simulink model "simulink_aocs_spin"  (R2023b)
settings: Solver=VariableStepAuto  StartTime=0.0  StopTime=10.0  RelTol=1e-3
values from neighbouring files (symbols this model uses):
  A0 = [1 0 0; 0 0 1; 0 -1 0]*[0 0 1; 0 1 0; -1 0 0]    [planetary_phase_script.m]    (also in script_aocs.m = [0 0 1; 0 1 0; -1 0 0]; script_jupiter.m; simulation_inner1.m = A_b_n(:,:,end); srp_interplanetary.m = A_b_n(:,:,end))
  braccio_x = 2.7    [planetary_phase_script.m]    (also in script_aocs.m; script_jupiter.m; simulation_inner1.m; srp_interplanetary.m)
  braccio_y = 2.7    [planetary_phase_script.m]    (also in script_aocs.m; script_jupiter.m; simulation_inner1.m; srp_interplanetary.m)
  braccio_z = 3.2    [planetary_phase_script.m]    (also in script_aocs.m; script_jupiter.m; simulation_inner1.m; srp_interplanetary.m)
  gain_alphas = [-1000; -1000; -10]    [planetary_phase_script.m]    (also in script_aocs.m = -90; script_jupiter.m; simulation_inner1.m = [-100 -100 -1]'; srp_interplanetary.m = [-100 -100 -1]')
  gain_omega = -1    [planetary_phase_script.m]    (also in script_aocs.m = -9500; script_jupiter.m; simulation_inner1.m = -950; srp_interplanetary.m = -950)
  I = diag([11245.08 10044.71 17593.63])    [planetary_phase_script.m]    (also in script_aocs.m = [11245.08 0 0; 0 10044.71 0; 0 0 17593.63]; script_jupiter.m; simulation_inner1.m = [11245.08 0 0; 0 10044.71 0; 0 0 17593.63]; srp_interplanetary.m = [11245.08 0 0; 0 10044.71 0; 0 0 17593.63])
  I_inv = inv(I)    [planetary_phase_script.m]    (also in script_aocs.m; script_jupiter.m; simulation_inner1.m; srp_interplanetary.m)
  spin_fin = spin(j,2) * 2*pi/60    [script_aocs.m]
  t_s = 1    [script_aocs.m]    (also in simulation_inner1.m; srp_interplanetary.m)
  toll = deg2rad(15)    [planetary_phase_script.m]    (also in script_aocs.m; script_jupiter.m; simulation_inner1.m; srp_interplanetary.m)
  w0 = [0 0 n]    [planetary_phase_script.m]    (also in script_aocs.m = [0 0 spin_0]; script_jupiter.m; simulation_inner1.m = w(:,end); srp_interplanetary.m = w(:,end))
libraries: simulink x3, matrix_library x1
settings Model: SimulationMode=accelerator  Creator=paolo  LastModifiedBy=paolo

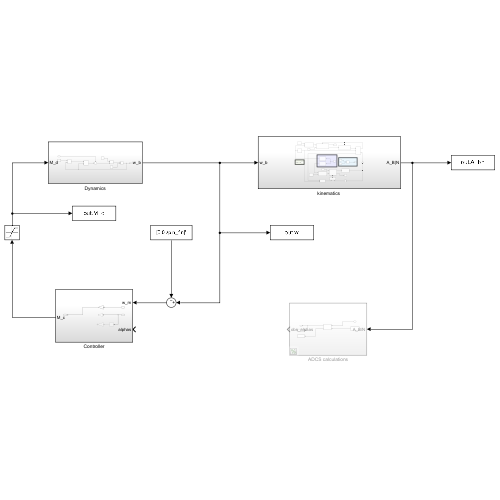
[thumbnail: Simulink's stored preview of the top-level diagram]
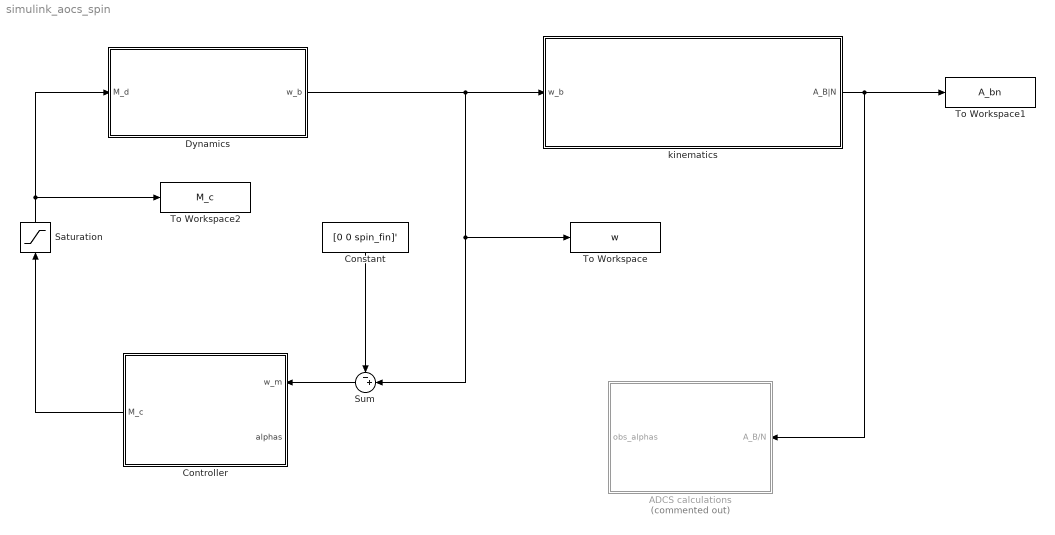
== system simulink_aocs_spin ==
  ADCS calculations : Subsystem  Commented=on
  Constant : Constant  Value=[0 0 spin_fin]'
  Controller : Subsystem
  Dynamics : Subsystem
  Saturation : Saturate  UpperLimit=5*[braccio_x braccio_y braccio_z]'  LowerLimit=-5*[braccio_x braccio_y braccio_z]'
  Sum : Sum  Inputs=-+|
  To Workspace : ToWorkspace  VariableName=w  SampleTime=-1
  To Workspace1 : ToWorkspace  VariableName=A_bn  SampleTime=-1
  To Workspace2 : ToWorkspace  VariableName=M_c  SampleTime=-1
  "kinematics " : Subsystem
  wires:
  "kinematics "/1(A_B|N) -> To Workspace1/1, ADCS calculations/1(" A_B/N")
  Saturation/1 -> Dynamics/1(M_d), To Workspace2/1
  Sum/1 -> Controller/1(w_m)
  Constant/1 -> Sum/1
  Dynamics/1(w_b) -> "kinematics "/1(w_b), To Workspace/1, Sum/2
  Controller/1(M_c) -> Saturation/1

== system simulink_aocs_spin/ADCS calculations ==
  " A_B/N" : Inport
  Error determination1 : Subsystem
  To Workspace10 : ToWorkspace  VariableName=alphas  SampleTime=-1
  To Workspace2 : ToWorkspace  VariableName=error_matrix  SampleTime=-1
  targeting attitude : Subsystem
  obs_alphas : Outport
  wires:
  Error determination1/2(Error Matrix) -> To Workspace2/1
  Error determination1/1(alphas) -> To Workspace10/1, obs_alphas/1
  targeting attitude/1(target) -> Error determination1/2(target)
  " A_B/N"/1 -> Error determination1/1(sensed A_b|n)

== system simulink_aocs_spin/Controller ==
  w_m : Inport
  alphas : Inport  Port=2
  Gain1 : Gain  Commented=on  Gain=-0.0075
  Gain3 : Gain  Gain=gain_omega
  Gain4 : Gain  Commented=on  Gain=gain_alphas
  Integrator : Integrator  Commented=on
  M_c : Outport
  wires:
  Gain3/1 -> M_c/1
  w_m/1 -> Gain3/1  "w_m"
  alphas/1 -> Integrator/1, Gain4/1  "alphas"
  Integrator/1 -> Gain1/1

== system simulink_aocs_spin/Dynamics ==
  M_d : Inport
  Add : Sum  Inputs=++|
  Constant : Constant  Value=I_inv
  Constant1 : Constant  Value=I
  Constant2 : Constant  Value=w0
  Cross Product : matrix_library/Cross Product
  Integrator : Integrator  InitialConditionSource=external
  Product3 : Product  Multiplication=Matrix(*)
  Product4 : Product  Multiplication=Matrix(*)
  w_b : Outport
  wires:
  Constant2/1 -> Integrator/2
  Integrator/1 -> Cross Product/2, Product3/2, w_b/1
  Constant1/1 -> Product3/1
  Product3/1 -> Cross Product/1
  Cross Product/1 -> Add/2
  Constant/1 -> Product4/1
  Product4/1 -> Integrator/1
  Add/1 -> Product4/2
  M_d/1 -> Add/1

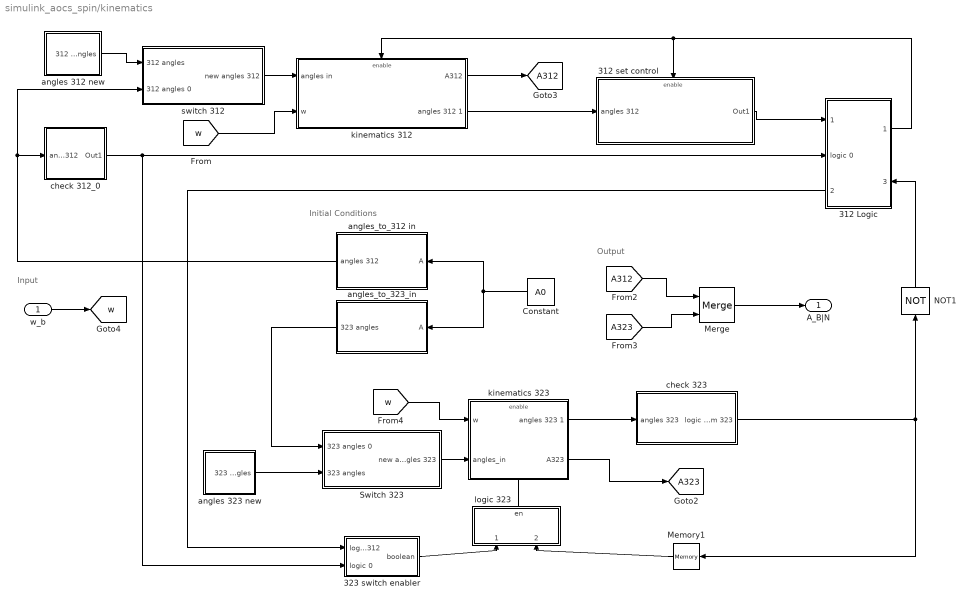
== system simulink_aocs_spin/kinematics  ==
  note: Initial Conditions
  note: Input
  note: Output
  w_b : Inport
  312 Logic : Subsystem
      settings: PortSchema="{\"entries\":[{\"content\":{\"sides\":[{\"content\":{\"connectorIds\":[\"In1\",\"In2\",\"Out2\"]},\"type\":\"ConnectorPlacement.EquallySpacedRectSide\",\"uuid\":\"bbe9512c-7163-4fef-b9d1-43cb9aeff445\"},{\"content\":{\"connectorIds\":[\"Out1\",\"In3\"],\"side\":\"RIGHT\"},\"type\":\"ConnectorPlacement.EquallySpacedRectSide\",\"uuid\":\"277562d8-09f7-4de0-8511-9dc3831eb0dd\"},{\"content\":{\"side\":\"TOP\"},\"type\":\"ConnectorPlacement.EquallySpacedRectSide\",\"uuid\":\"e92148c3-32f1-4524-99fb-140743ec3546\"},{\"content\":{\"side\":\"BOTTOM\"},\"type\":\"ConnectorPlacement.EquallySpacedRectSide\",\"uuid\":\"83e80a71-3551-431b-aa8d-7f5ff14dcfcb\"}]},\"type\":\"ConnectorPlacement.EquallySpacedConnector\",\"uuid\":\"c3d5c0ca-8775-4917-b094-b0cdc270e969\"}],\"packageUris\":[\"http://schema.mathworks.com/mf0/Connector/R2020b\"],\"version\":\"1.0\"}"
  312 set control : Subsystem
  323 switch enabler : Subsystem
  Constant : Constant  Value=A0
  Memory1 : Memory
  Merge : Merge
  NOT1 : Logic  Operator=NOT  IconShape=distinctive  AllPortsSameDT=off  OutDataTypeStr=boolean
  Switch 323 : Subsystem
  angles 312 new : Subsystem
  angles 323 new : Subsystem
  angles_to_312 in : Subsystem
  angles_to_323_in : Subsystem
  check 312_0 : Subsystem
      settings: PortSchema="{\"entries\":[{\"content\":{\"sides\":[{\"content\":{},\"type\":\"ConnectorPlacement.EquallySpacedRectSide\",\"uuid\":\"ce510fac-c30a-4239-a3ca-34d3b3a25917\"},{\"content\":{\"side\":\"RIGHT\"},\"type\":\"ConnectorPlacement.EquallySpacedRectSide\",\"uuid\":\"eef8e0af-d591-4c9d-a699-4633d685d136\"},{\"content\":{\"connectorIds\":[\"Out1\"],\"side\":\"TOP\"},\"type\":\"ConnectorPlacement.EquallySpacedRectSide\",\"uuid\":\"fcaa08d0-a3a1-4dce-b64a-8b5dfd06733d\"},{\"content\":{\"connectorIds\":[\"In1\"],\"side\":\"BOTTOM\"},\"type\":\"ConnectorPlacement.EquallySpacedRectSide\",\"uuid\":\"e9ea2ab9-2ba0-4219-9d61-f42bbc501f13\"}]},\"type\":\"ConnectorPlacement.EquallySpacedConnector\",\"uuid\":\"4537d4ba-38a8-4a93-90f3-8d5d5085984b\"}],\"packageUris\":[\"http://schema.mathworks.com/mf0/Connector/R2020b\"],\"version\":\"1.0\"}"
  check 323 : Subsystem
      settings: PortSchema="{\"entries\":[{\"content\":{\"sides\":[{\"content\":{},\"type\":\"ConnectorPlacement.EquallySpacedRectSide\",\"uuid\":\"ce510fac-c30a-4239-a3ca-34d3b3a25917\"},{\"content\":{\"side\":\"RIGHT\"},\"type\":\"ConnectorPlacement.EquallySpacedRectSide\",\"uuid\":\"eef8e0af-d591-4c9d-a699-4633d685d136\"},{\"content\":{\"connectorIds\":[\"Out1\"],\"side\":\"TOP\"},\"type\":\"ConnectorPlacement.EquallySpacedRectSide\",\"uuid\":\"fcaa08d0-a3a1-4dce-b64a-8b5dfd06733d\"},{\"content\":{\"connectorIds\":[\"In1\"],\"side\":\"BOTTOM\"},\"type\":\"ConnectorPlacement.EquallySpacedRectSide\",\"uuid\":\"e9ea2ab9-2ba0-4219-9d61-f42bbc501f13\"}]},\"type\":\"ConnectorPlacement.EquallySpacedConnector\",\"uuid\":\"4537d4ba-38a8-4a93-90f3-8d5d5085984b\"}],\"packageUris\":[\"http://schema.mathworks.com/mf0/Connector/R2020b\"],\"version\":\"1.0\"}"
  kinematics 312 : Subsystem
  kinematics 323 : Subsystem
  logic 323 : Subsystem
  switch 312 : Subsystem
  A_B|N : Outport
  tag scope: A312=global, A323=global, w=global
  wires:
  kinematics 323/2(A323) -> [A323]
  Constant/1 -> angles_to_323_in/1(A), angles_to_312 in/1(A)
  323 switch enabler/1(boolean) -> logic 323/1(boolean from 312)
  logic 323/1(en) -> kinematics 323/Enable
  kinematics 312/2(angles 312 1) -> 312 set control/1(angles 312)
  check 312_0/1(Out1) -> 323 switch enabler/2(logic 0), 312 Logic/2(logic 0)
  [w] -> kinematics 323/1(w)
  angles_to_312 in/1(angles 312) -> switch 312/2(312 angles 0), check 312_0/1(angles 312)
  Memory1/1 -> logic 323/2(boolean from 323)
  w_b/1 -> [w]
  kinematics 323/1(angles 323 1) -> check 323/1(angles 323)
  kinematics 312/1(A312) -> [A312]
  switch 312/1(new angles 312) -> kinematics 312/1(angles in)
  Merge/1 -> A_B|N/1
  Switch 323/1(new angles 323) -> kinematics 323/2(angles_in)
  check 323/1(logic from 323) -> NOT1/1, Memory1/1
  angles 323 new/1(323 angles) -> Switch 323/2(323 angles)
  angles 312 new/1(312 angles) -> switch 312/1(312 angles)
  [w] -> kinematics 312/2(w)
  angles_to_323_in/1(323 angles) -> Switch 323/1(323 angles 0)
  [A323] -> Merge/2
  [A312] -> Merge/1
  312 Logic/1(logic to 312) -> kinematics 312/Enable, 312 set control/Enable
  312 set control/1(Out1) -> 312 Logic/1(logic from 312)
  NOT1/1 -> 312 Logic/3(logic from 323)
  312 Logic/2(logic to 323) -> 323 switch enabler/1(logic from 312)

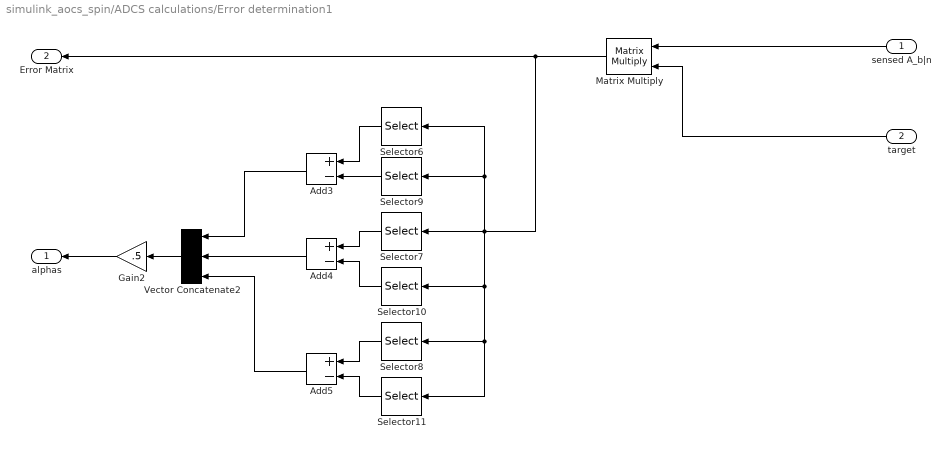
== system simulink_aocs_spin/ADCS calculations/Error determination1 ==
  sensed A_b|n : Inport
  target : Inport  Port=2
  Add3 : Sum  Inputs=+-
  Add4 : Sum  Inputs=+-
  Add5 : Sum  Inputs=+-
  Gain2 : Gain  Gain=.5
  Matrix Multiply : Product  Multiplication=Matrix(*)
  Selector10 : Selector  NumberOfDimensions=2  InputPortWidth=3  IndexOptions=Index vector (dialog),Index vector (dialog)  Indices=1,3  OutputSizes=1,1
  Selector11 : Selector  NumberOfDimensions=2  InputPortWidth=3  IndexOptions=Index vector (dialog),Index vector (dialog)  Indices=2,1  OutputSizes=1,1
  Selector6 : Selector  NumberOfDimensions=2  InputPortWidth=3  IndexOptions=Index vector (dialog),Index vector (dialog)  Indices=2,3  OutputSizes=1,1
  Selector7 : Selector  NumberOfDimensions=2  InputPortWidth=3  IndexOptions=Index vector (dialog),Index vector (dialog)  Indices=3,1  OutputSizes=1,1
  Selector8 : Selector  NumberOfDimensions=2  InputPortWidth=3  IndexOptions=Index vector (dialog),Index vector (dialog)  Indices=1,2  OutputSizes=1,1
  Selector9 : Selector  NumberOfDimensions=2  InputPortWidth=3  IndexOptions=Index vector (dialog),Index vector (dialog)  Indices=3,2  OutputSizes=1,1
  Vector Concatenate2 : Concatenate  NumInputs=3
  alphas : Outport
  Error Matrix : Outport  Port=2
  wires:
  Gain2/1 -> alphas/1
  Add4/1 -> Vector Concatenate2/2
  Selector6/1 -> Add3/1
  Selector11/1 -> Add5/2
  Vector Concatenate2/1 -> Gain2/1
  Add3/1 -> Vector Concatenate2/1
  Selector7/1 -> Add4/1
  Selector10/1 -> Add4/2
  Matrix Multiply/1 -> Selector7/1, Selector10/1, Selector11/1, Selector8/1, Selector9/1, Selector6/1, Error Matrix/1
  Selector8/1 -> Add5/1
  Selector9/1 -> Add3/2
  Add5/1 -> Vector Concatenate2/3
  sensed A_b|n/1 -> Matrix Multiply/1
  target/1 -> Matrix Multiply/2

== system simulink_aocs_spin/ADCS calculations/targeting attitude ==
  Constant1 : Constant  Value=[0 0 -1; 0 1 0; 1 0 0]
  Matrix Multiply : Product  Multiplication=Matrix(*)
  Rotation matrix n : Subsystem
  target : Outport
  wires:
  Matrix Multiply/1 -> target/1
  Constant1/1 -> Matrix Multiply/1
  Rotation matrix n/1(Target matrix) -> Matrix Multiply/2

== system simulink_aocs_spin/kinematics /312 Logic ==
  logic from 312 : Inport
  logic 0 : Inport  Port=2
  logic from 323 : Inport  Port=3
  Memory : Memory  InheritSampleTime=on
  Subsystem3 : Subsystem
  switch enabler 312 : Subsystem
  logic to 312 : Outport
  logic to 323 : Outport  Port=2
  wires:
  Subsystem3/1(Out1) -> Memory/1
  logic 0/1 -> switch enabler 312/2(In2)
  Memory/1 -> switch enabler 312/1(In1), Subsystem3/3(In3), logic to 323/1
  logic from 323/1 -> Subsystem3/2(In2)
  switch enabler 312/1(Out1) -> logic to 312/1
  logic from 312/1 -> Subsystem3/1(In1)

== system simulink_aocs_spin/kinematics /312 set control ==
  angles 312 : Inport
  Enable : EnablePort
  Check Static Range : simulink/Model Verification/Check  Static Range  Description=-pi/2+toll <= u <= pi/2 - toll  max=pi/2 - toll  max_included=on  min=-pi/2+toll  min_included=on  enabled=off  stopWhenAssertionFail=off  export=on  icon=graphic
  Selector : Selector  InputPortWidth=3  IndexOptions=Index vector (dialog)  Indices=2  OutputSizes=1
  Out1 : Outport
  wires:
  Check Static Range/1 -> Out1/1
  angles 312/1 -> Selector/1
  Selector/1 -> Check Static Range/1

== system simulink_aocs_spin/kinematics /323 switch enabler ==
  logic from 312 : Inport
  logic 0 : Inport  Port=2
  Clock2 : Clock
  NOT : Logic  Operator=NOT  IconShape=distinctive  AllPortsSameDT=off  OutDataTypeStr=boolean
  Switch2 : Switch  Criteria=u2 > Threshold  SaturateOnIntegerOverflow=off  InputSameDT=off
  boolean : Outport
  wires:
  Switch2/1 -> NOT/1
  logic 0/1 -> Switch2/3
  Clock2/1 -> Switch2/2
  logic from 312/1 -> Switch2/1
  NOT/1 -> boolean/1

== system simulink_aocs_spin/kinematics /Switch 323 ==
  323 angles 0 : Inport
  323 angles : Inport  Port=2
  Clock3 : Clock
  Switch3 : Switch  Criteria=u2 > Threshold  SaturateOnIntegerOverflow=off  InputSameDT=off
  new angles 323 : Outport
  wires:
  Clock3/1 -> Switch3/2
  323 angles 0/1 -> Switch3/3
  323 angles/1 -> Switch3/1
  Switch3/1 -> new angles 323/1

== system simulink_aocs_spin/kinematics /angles 312 new ==
  A323 matrix : Subsystem
  angles_to_312 : Subsystem
  312 angles : Outport
  wires:
  [phi323] -> A323 matrix/1(phi)
  [theta323] -> A323 matrix/2(theta)
  [psi323] -> A323 matrix/3(psi)
  angles_to_312/1(312 angles) -> 312 angles/1
  A323 matrix/1(A323) -> angles_to_312/1(A323)

== system simulink_aocs_spin/kinematics /angles 323 new ==
  Rotation 312 matrix2 : Subsystem
  angles_to_323 : Subsystem
  323 angles : Outport
  wires:
  [theta312] -> Rotation 312 matrix2/2(theta)
  [psi_312] -> Rotation 312 matrix2/3(psi)
  Rotation 312 matrix2/1(A312) -> angles_to_323/1(A312)
  [phi312] -> Rotation 312 matrix2/1(phi)
  angles_to_323/1(323 angles) -> 323 angles/1

== system simulink_aocs_spin/kinematics /angles_to_312 in ==
  A : Inport
  Asin : Trigonometry  Operator=asin
  Atan1 : Trigonometry  Operator=atan2
  Atan2 : Trigonometry  Operator=atan2
  Gain : Gain  Gain=-1
  Gain1 : Gain  Gain=-1
  Mux : Mux  Inputs=3
  Selector : Selector  NumberOfDimensions=2  InputPortWidth=3  IndexOptions=Index vector (dialog),Index vector (dialog)  Indices=2,1  OutputSizes=1,1
  Selector1 : Selector  NumberOfDimensions=2  InputPortWidth=3  IndexOptions=Index vector (dialog),Index vector (dialog)  Indices=2,2  OutputSizes=1,1
  Selector2 : Selector  NumberOfDimensions=2  InputPortWidth=3  IndexOptions=Index vector (dialog),Index vector (dialog)  Indices=2,3  OutputSizes=1,1
  Selector3 : Selector  NumberOfDimensions=2  InputPortWidth=3  IndexOptions=Index vector (dialog),Index vector (dialog)  Indices=1,3  OutputSizes=1,1
  Selector4 : Selector  NumberOfDimensions=2  InputPortWidth=3  IndexOptions=Index vector (dialog),Index vector (dialog)  Indices=3,3  OutputSizes=1,1
  angles 312 : Outport
  wires:
  Selector/1 -> Gain/1
  Gain/1 -> Atan2/1
  Selector1/1 -> Atan2/2
  Selector2/1 -> Asin/1
  Atan2/1 -> Mux/1
  Asin/1 -> Mux/2
  Mux/1 -> angles 312/1
  A/1 -> Selector3/1, Selector4/1, Selector2/1, Selector/1, Selector1/1
  Selector3/1 -> Gain1/1
  Gain1/1 -> Atan1/1
  Selector4/1 -> Atan1/2
  Atan1/1 -> Mux/3

== system simulink_aocs_spin/kinematics /angles_to_323_in ==
  A : Inport
  Asin : Trigonometry  Operator=acos
  Atan1 : Trigonometry  Operator=atan2
  Atan2 : Trigonometry  Operator=atan2
  Gain2 : Gain  Gain=-1
  Mux : Mux  Inputs=3
  Selector : Selector  NumberOfDimensions=2  InputPortWidth=3  IndexOptions=Index vector (dialog),Index vector (dialog)  Indices=3,2  OutputSizes=1,1
  Selector1 : Selector  NumberOfDimensions=2  InputPortWidth=3  IndexOptions=Index vector (dialog),Index vector (dialog)  Indices=3,1  OutputSizes=1,1
  Selector2 : Selector  NumberOfDimensions=2  InputPortWidth=3  IndexOptions=Index vector (dialog),Index vector (dialog)  Indices=3,3  OutputSizes=1,1
  Selector3 : Selector  NumberOfDimensions=2  InputPortWidth=3  IndexOptions=Index vector (dialog),Index vector (dialog)  Indices=2,3  OutputSizes=1,1
  Selector4 : Selector  NumberOfDimensions=2  InputPortWidth=3  IndexOptions=Index vector (dialog),Index vector (dialog)  Indices=1,3  OutputSizes=1,1
  323 angles : Outport
  wires:
  Gain2/1 -> Atan1/2
  Selector1/1 -> Atan2/2
  Selector2/1 -> Asin/1
  Selector/1 -> Atan2/1
  A/1 -> Selector2/1, Selector4/1, Selector3/1, Selector1/1, Selector/1
  Atan1/1 -> Mux/3
  Atan2/1 -> Mux/1
  Selector4/1 -> Gain2/1
  Selector3/1 -> Atan1/1
  Asin/1 -> Mux/2
  Mux/1 -> 323 angles/1

== system simulink_aocs_spin/kinematics /check 312_0 ==
  angles 312 : Inport
  Check Static Range : simulink/Model Verification/Check  Static Range  Description=-pi/2+toll <= u <= pi/2 - toll  max=pi/2 - toll  max_included=on  min=-pi/2+toll  min_included=on  enabled=off  stopWhenAssertionFail=off  export=on  icon=graphic
  Data Type Conversion : DataTypeConversion  OutDataTypeStr=boolean  SaturateOnIntegerOverflow=off  RndMeth=Floor
  Selector : Selector  InputPortWidth=3  IndexOptions=Index vector (dialog)  Indices=[2]  OutputSizes=1
  Out1 : Outport
  wires:
  angles 312/1 -> Selector/1
  Selector/1 -> Check Static Range/1
  Check Static Range/1 -> Data Type Conversion/1
  Data Type Conversion/1 -> Out1/1

== system simulink_aocs_spin/kinematics /check 323 ==
  angles 323 : Inport
  Check Static Range : simulink/Model Verification/Check  Static Range  Description=toll <= u <= pi - toll  max=pi - toll  max_included=on  min=toll  min_included=on  enabled=off  stopWhenAssertionFail=off  export=on  icon=graphic
  Selector : Selector  InputPortWidth=3  IndexOptions=Index vector (dialog)  Indices=2  OutputSizes=1
  logic from 323 : Outport
  wires:
  Check Static Range/1 -> logic from 323/1
  Selector/1 -> Check Static Range/1
  angles 323/1 -> Selector/1

== system simulink_aocs_spin/kinematics /kinematics 312 ==
  angles in : Inport
  w : Inport  Port=2
  Enable : EnablePort  StatesWhenEnabling=reset  ShowOutputPort=on
  Kinematics 312 : Subsystem
      settings: PortSchema="{\"entries\":[{\"content\":{\"sides\":[{\"content\":{\"connectorIds\":[\"In1\",\"In2\"]},\"type\":\"ConnectorPlacement.EquallySpacedRectSide\",\"uuid\":\"4fd6e809-7da2-4d51-96c7-4627657bb0a7\"},{\"content\":{\"connectorIds\":[\"Out1\"],\"side\":\"RIGHT\"},\"type\":\"ConnectorPlacement.EquallySpacedRectSide\",\"uuid\":\"c66e7720-5f48-4c1c-aaff-2c7b43e45843\"},{\"content\":{\"connectorIds\":[\"In3\"],\"side\":\"TOP\"},\"type\":\"ConnectorPlacement.EquallySpacedRectSide\",\"uuid\":\"5add9d35-dacd-40f3-b2c8-04b7016dc331\"}]},\"type\":\"ConnectorPlacement.EquallySpacedConnector\",\"uuid\":\"f50f8b24-6836-47e2-b898-11b49150a1de\"}],\"packageUris\":[\"http://schema.mathworks.com/mf0/Connector/R2020b\"],\"version\":\"1.0\"}"
  Rotation 312 matrix1 : Subsystem
  A312 : Outport
  angles 312 1 : Outport  Port=2
  wires:
  Rotation 312 matrix1/1(A312) -> A312/1
  Kinematics 312/1(angles) -> Rotation 312 matrix1/1(angles), angles 312 1/1
  angles in/1 -> Kinematics 312/2(angles in)
  w/1 -> Kinematics 312/1(w)
  Enable/1 -> Kinematics 312/3(enabler)

== system simulink_aocs_spin/kinematics /kinematics 323 ==
  w : Inport
  angles_in : Inport  Port=2
  Enable : EnablePort  StatesWhenEnabling=reset  ShowOutputPort=on
  " kinematics 323" : Subsystem
      settings: PortSchema="{\"entries\":[{\"content\":{\"sides\":[{\"content\":{\"connectorIds\":[\"In1\",\"In2\"]},\"type\":\"ConnectorPlacement.EquallySpacedRectSide\",\"uuid\":\"4fd6e809-7da2-4d51-96c7-4627657bb0a7\"},{\"content\":{\"connectorIds\":[\"Out1\"],\"side\":\"RIGHT\"},\"type\":\"ConnectorPlacement.EquallySpacedRectSide\",\"uuid\":\"c66e7720-5f48-4c1c-aaff-2c7b43e45843\"},{\"content\":{\"connectorIds\":[\"In3\"],\"side\":\"TOP\"},\"type\":\"ConnectorPlacement.EquallySpacedRectSide\",\"uuid\":\"5add9d35-dacd-40f3-b2c8-04b7016dc331\"}]},\"type\":\"ConnectorPlacement.EquallySpacedConnector\",\"uuid\":\"f50f8b24-6836-47e2-b898-11b49150a1de\"}],\"packageUris\":[\"http://schema.mathworks.com/mf0/Connector/R2020b\"],\"version\":\"1.0\"}"
  A323 matrix1 : Subsystem
  angles 323 1 : Outport
  A323 : Outport  Port=2
  wires:
  angles_in/1 -> " kinematics 323"/1(angles_in)
  w/1 -> " kinematics 323"/2(w)
  A323 matrix1/1(A323) -> A323/1
  " kinematics 323"/1(angles) -> angles 323 1/1, A323 matrix1/1(angles)
  Enable/1 -> " kinematics 323"/3(enable)

== system simulink_aocs_spin/kinematics /logic 323 ==
  boolean from 312 : Inport
  boolean from 323 : Inport  Port=2
  AND : Logic  IconShape=distinctive  AllPortsSameDT=off  OutDataTypeStr=boolean
  Clock3 : Clock
  Memory : Memory
  Subsystem4 : Subsystem
  Switch3 : Switch  Criteria=u2 > Threshold  SaturateOnIntegerOverflow=off  InputSameDT=off
  en : Outport
  wires:
  Switch3/1 -> en/1, Memory/1
  Clock3/1 -> Switch3/2
  boolean from 323/1 -> Subsystem4/1(In2), AND/1
  boolean from 312/1 -> Subsystem4/3(In4), Switch3/3, AND/2
  Subsystem4/1(Out1) -> Switch3/1
  AND/1 -> Subsystem4/2(In1)
  Memory/1 -> Subsystem4/4(In3)

== system simulink_aocs_spin/kinematics /switch 312 ==
  312 angles : Inport
  312 angles 0 : Inport  Port=2
  Clock : Clock
  Switch : Switch  Criteria=u2 > Threshold  SaturateOnIntegerOverflow=off  InputSameDT=off
  new angles 312 : Outport
  wires:
  Switch/1 -> new angles 312/1
  312 angles/1 -> Switch/1
  Clock/1 -> Switch/2
  312 angles 0/1 -> Switch/3

== system simulink_aocs_spin/ADCS calculations/targeting attitude/Rotation matrix n ==
  Constant : Constant  Value=0
  Constant1 : Constant
  Cos : Trigonometry  Operator=cos
  Digital Clock : DigitalClock  SampleTime=t_s
  Gain : Gain  Gain=spin_fin
  Gain1 : Gain
  Gain2 : Gain  Gain=-1
  Sin : Trigonometry
  Target : Concatenate  NumInputs=3  Mode=Multidimensional array  ConcatenateDimension=2
  Vector Concatenate : Concatenate  NumInputs=3
  Vector Concatenate1 : Concatenate  NumInputs=3
  Vector Concatenate2 : Concatenate  NumInputs=3
  Target matrix : Outport
  wires:
  Vector Concatenate/1 -> Target/1
  Sin/1 -> Gain2/1, Gain1/1
  Cos/1 -> Vector Concatenate2/1, Vector Concatenate1/2
  Digital Clock/1 -> Gain/1
  Gain/1 -> Cos/1, Sin/1
  Constant/1 -> Vector Concatenate/1, Vector Concatenate2/3, Vector Concatenate1/3, Vector Concatenate/2
  Vector Concatenate2/1 -> Target/3
  Vector Concatenate1/1 -> Target/2
  Target/1 -> Target matrix/1
  Constant1/1 -> Vector Concatenate/3
  Gain1/1 -> Vector Concatenate1/1
  Gain2/1 -> Vector Concatenate2/2

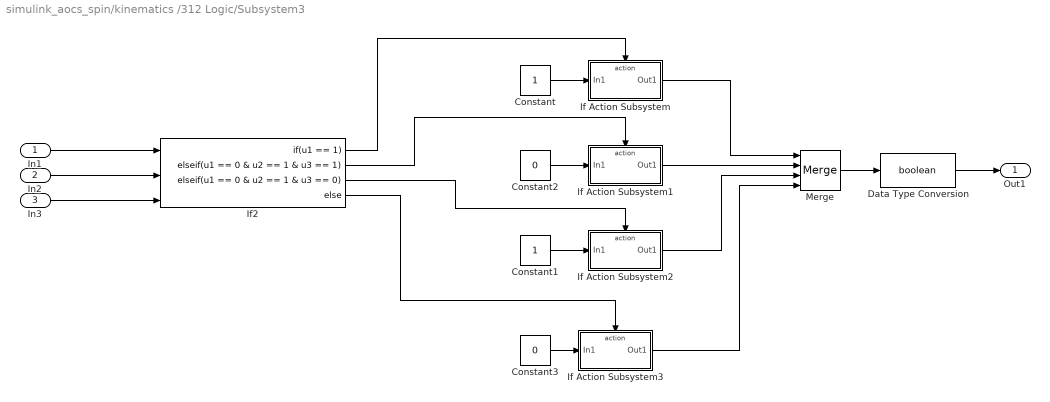
== system simulink_aocs_spin/kinematics /312 Logic/Subsystem3 ==
  In1 : Inport
  In2 : Inport  Port=2
  In3 : Inport  Port=3
  Constant : Constant
  Constant1 : Constant
  Constant2 : Constant  Value=0
  Constant3 : Constant  Value=0
  Data Type Conversion : DataTypeConversion  OutDataTypeStr=boolean  SaturateOnIntegerOverflow=off  RndMeth=Floor
  If Action Subsystem : Subsystem  TreatAsAtomicUnit=on
  If Action Subsystem1 : Subsystem  TreatAsAtomicUnit=on
  If Action Subsystem2 : Subsystem  TreatAsAtomicUnit=on
  If Action Subsystem3 : Subsystem  TreatAsAtomicUnit=on
  If2 : If  NumInputs=3  IfExpression=u1 == 1  ElseIfExpressions=u1 == 0 & u2 == 1 & u3 == 1, u1 == 0 & u2 == 1 & u3 == 0
  Merge : Merge  Inputs=4
  Out1 : Outport
  wires:
  In2/1 -> If2/2
  In1/1 -> If2/1
  In3/1 -> If2/3
  If2/1 -> If Action Subsystem/Action
  If2/2 -> If Action Subsystem1/Action
  If2/3 -> If Action Subsystem2/Action
  If2/4 -> If Action Subsystem3/Action
  Constant/1 -> If Action Subsystem/1(In1)
  Constant1/1 -> If Action Subsystem2/1(In1)
  Constant2/1 -> If Action Subsystem1/1(In1)
  Constant3/1 -> If Action Subsystem3/1(In1)
  If Action Subsystem/1(Out1) -> Merge/1
  If Action Subsystem1/1(Out1) -> Merge/2
  If Action Subsystem2/1(Out1) -> Merge/3
  If Action Subsystem3/1(Out1) -> Merge/4
  Merge/1 -> Data Type Conversion/1
  Data Type Conversion/1 -> Out1/1

== system simulink_aocs_spin/kinematics /312 Logic/switch enabler 312 ==
  In1 : Inport
  In2 : Inport  Port=2
  Clock1 : Clock
  Switch1 : Switch  Criteria=u2 > Threshold  SaturateOnIntegerOverflow=off  InputSameDT=off
  Out1 : Outport
  wires:
  In2/1 -> Switch1/3
  Clock1/1 -> Switch1/2
  In1/1 -> Switch1/1
  Switch1/1 -> Out1/1

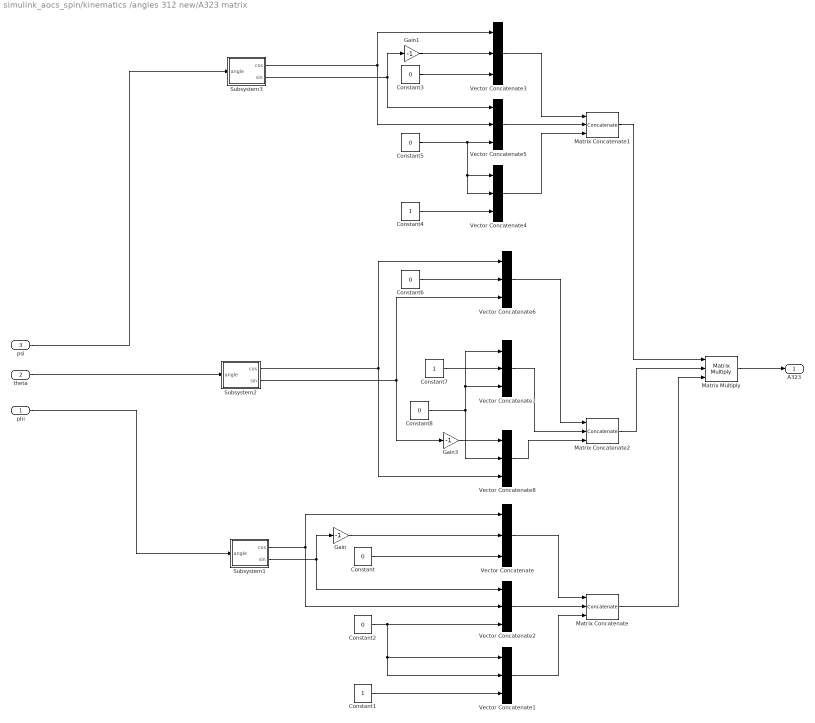
== system simulink_aocs_spin/kinematics /angles 312 new/A323 matrix ==
  phi : Inport
  theta : Inport  Port=2
  psi : Inport  Port=3
  Constant{,2..3,5..6,8} (6 alike) : Constant  Value=0
  Constant1 : Constant
  Constant4 : Constant
  Constant7 : Constant
  Gain : Gain  Gain=-1
  Gain1 : Gain  Gain=-1
  Gain3 : Gain  Gain=-1
  Matrix Concatenate : Concatenate  NumInputs=3  Mode=Multidimensional array  ConcatenateDimension=2
  Matrix Concatenate1 : Concatenate  NumInputs=3  Mode=Multidimensional array  ConcatenateDimension=2
  Matrix Concatenate2 : Concatenate  NumInputs=3  Mode=Multidimensional array  ConcatenateDimension=2
  Matrix Multiply : Product  Inputs=3  Multiplication=Matrix(*)
  Subsystem1 : Subsystem
  Subsystem2 : Subsystem
  Subsystem3 : Subsystem
  Vector Concatenate{,1..8} (9 alike) : Concatenate  NumInputs=3
  A323 : Outport
  wires:
  Subsystem1/2(sin) -> Gain/1, Vector Concatenate2/1
  Subsystem1/1(cos) -> Vector Concatenate2/2, Vector Concatenate/1
  Constant1/1 -> Vector Concatenate1/3
  Gain/1 -> Vector Concatenate/2
  Constant/1 -> Vector Concatenate/3
  Constant2/1 -> Vector Concatenate1/1, Vector Concatenate1/2, Vector Concatenate2/3
  Vector Concatenate/1 -> Matrix Concatenate/1
  Vector Concatenate2/1 -> Matrix Concatenate/2
  Vector Concatenate1/1 -> Matrix Concatenate/3
  Vector Concatenate4/1 -> Matrix Concatenate1/3
  Vector Concatenate5/1 -> Matrix Concatenate1/2
  Vector Concatenate3/1 -> Matrix Concatenate1/1
  Constant5/1 -> Vector Concatenate5/3, Vector Concatenate4/1, Vector Concatenate4/2
  Constant3/1 -> Vector Concatenate3/3
  Gain1/1 -> Vector Concatenate3/2
  Constant4/1 -> Vector Concatenate4/3
  Subsystem3/1(cos) -> Vector Concatenate3/1, Vector Concatenate5/2
  Subsystem3/2(sin) -> Vector Concatenate5/1, Gain1/1
  Matrix Concatenate2/1 -> Matrix Multiply/2
  Matrix Concatenate/1 -> Matrix Multiply/3
  Matrix Concatenate1/1 -> Matrix Multiply/1
  Matrix Multiply/1 -> A323/1
  Vector Concatenate6/1 -> Matrix Concatenate2/1
  Vector Concatenate7/1 -> Matrix Concatenate2/2
  Vector Concatenate8/1 -> Matrix Concatenate2/3
  Subsystem2/1(cos) -> Vector Concatenate8/3, Vector Concatenate6/1
  Constant6/1 -> Vector Concatenate6/2
  Subsystem2/2(sin) -> Vector Concatenate6/3, Gain3/1
  Constant7/1 -> Vector Concatenate7/2
  Constant8/1 -> Vector Concatenate7/1, Vector Concatenate7/3, Vector Concatenate8/2
  Gain3/1 -> Vector Concatenate8/1
  psi/1 -> Subsystem3/1(angle)
  theta/1 -> Subsystem2/1(angle)
  phi/1 -> Subsystem1/1(angle)

== system simulink_aocs_spin/kinematics /angles 312 new/angles_to_312 ==
  A323 : Inport
  Asin : Trigonometry  Operator=asin
  Atan1 : Trigonometry  Operator=atan2
  Atan2 : Trigonometry  Operator=atan2
  Gain : Gain  Gain=-1
  Gain1 : Gain  Gain=-1
  Mux : Mux  Inputs=3
  Selector : Selector  NumberOfDimensions=2  InputPortWidth=3  IndexOptions=Index vector (dialog),Index vector (dialog)  Indices=2,1  OutputSizes=1,1
  Selector1 : Selector  NumberOfDimensions=2  InputPortWidth=3  IndexOptions=Index vector (dialog),Index vector (dialog)  Indices=2,2  OutputSizes=1,1
  Selector2 : Selector  NumberOfDimensions=2  InputPortWidth=3  IndexOptions=Index vector (dialog),Index vector (dialog)  Indices=2,3  OutputSizes=1,1
  Selector3 : Selector  NumberOfDimensions=2  InputPortWidth=3  IndexOptions=Index vector (dialog),Index vector (dialog)  Indices=1,3  OutputSizes=1,1
  Selector4 : Selector  NumberOfDimensions=2  InputPortWidth=3  IndexOptions=Index vector (dialog),Index vector (dialog)  Indices=3,3  OutputSizes=1,1
  312 angles : Outport
  wires:
  Selector/1 -> Gain/1
  Gain/1 -> Atan2/1
  Selector1/1 -> Atan2/2
  Selector2/1 -> Asin/1
  Atan2/1 -> Mux/1
  Asin/1 -> Mux/2
  Mux/1 -> 312 angles/1
  A323/1 -> Selector/1, Selector1/1, Selector3/1, Selector4/1, Selector2/1
  Selector3/1 -> Gain1/1
  Gain1/1 -> Atan1/1
  Selector4/1 -> Atan1/2
  Atan1/1 -> Mux/3

== system simulink_aocs_spin/kinematics /angles 323 new/Rotation 312 matrix2 ==
  phi : Inport
  theta : Inport  Port=2
  psi : Inport  Port=3
  A312 conc : Concatenate  NumInputs=3  Mode=Multidimensional array  ConcatenateDimension=2
  Subsystem : Subsystem
  Subsystem1 : Subsystem
  Subsystem2 : Subsystem
  column 1 : Subsystem
  column 2 : Subsystem
  column 3 : Subsystem
  A312 : Outport
  wires:
  A312 conc/1 -> A312/1
  Subsystem/1(cos) -> column 2/1(phi), column 1/1(phi)
  column 3/1(Out1) -> A312 conc/3
  column 1/1(Out1) -> A312 conc/1
  Subsystem2/2(sin) -> column 3/4(psi2), column 2/6(psi2), column 1/6(psi2)
  column 2/1(Out1) -> A312 conc/2
  Subsystem2/1(cos) -> column 3/3(psi), column 1/5(psi), column 2/5(psi)
  Subsystem1/2(sin) -> column 2/4(theta2), column 1/4(theta2), column 3/2(theta2)
  Subsystem/2(sin) -> column 2/2(phi2), column 1/2(phi2)
  Subsystem1/1(cos) -> column 1/3(theta), column 3/1(theta), column 2/3(theta)
  phi/1 -> Subsystem/1(angle)
  theta/1 -> Subsystem1/1(angle)
  psi/1 -> Subsystem2/1(angle)

== system simulink_aocs_spin/kinematics /angles 323 new/angles_to_323 ==
  A312 : Inport
  Asin : Trigonometry  Operator=acos
  Atan1 : Trigonometry  Operator=atan2
  Atan2 : Trigonometry  Operator=atan2
  Gain2 : Gain  Gain=-1
  Mux : Mux  Inputs=3
  Selector : Selector  NumberOfDimensions=2  InputPortWidth=3  IndexOptions=Index vector (dialog),Index vector (dialog)  Indices=3,2  OutputSizes=1,1
  Selector1 : Selector  NumberOfDimensions=2  InputPortWidth=3  IndexOptions=Index vector (dialog),Index vector (dialog)  Indices=3,1  OutputSizes=1,1
  Selector2 : Selector  NumberOfDimensions=2  InputPortWidth=3  IndexOptions=Index vector (dialog),Index vector (dialog)  Indices=3,3  OutputSizes=1,1
  Selector3 : Selector  NumberOfDimensions=2  InputPortWidth=3  IndexOptions=Index vector (dialog),Index vector (dialog)  Indices=2,3  OutputSizes=1,1
  Selector4 : Selector  NumberOfDimensions=2  InputPortWidth=3  IndexOptions=Index vector (dialog),Index vector (dialog)  Indices=1,3  OutputSizes=1,1
  323 angles : Outport
  wires:
  Mux/1 -> 323 angles/1
  Asin/1 -> Mux/2
  Selector3/1 -> Atan1/1
  Selector4/1 -> Gain2/1
  Atan2/1 -> Mux/1
  Atan1/1 -> Mux/3
  A312/1 -> Selector/1, Selector1/1, Selector3/1, Selector4/1, Selector2/1
  Selector/1 -> Atan2/1
  Selector2/1 -> Asin/1
  Selector1/1 -> Atan2/2
  Gain2/1 -> Atan1/2

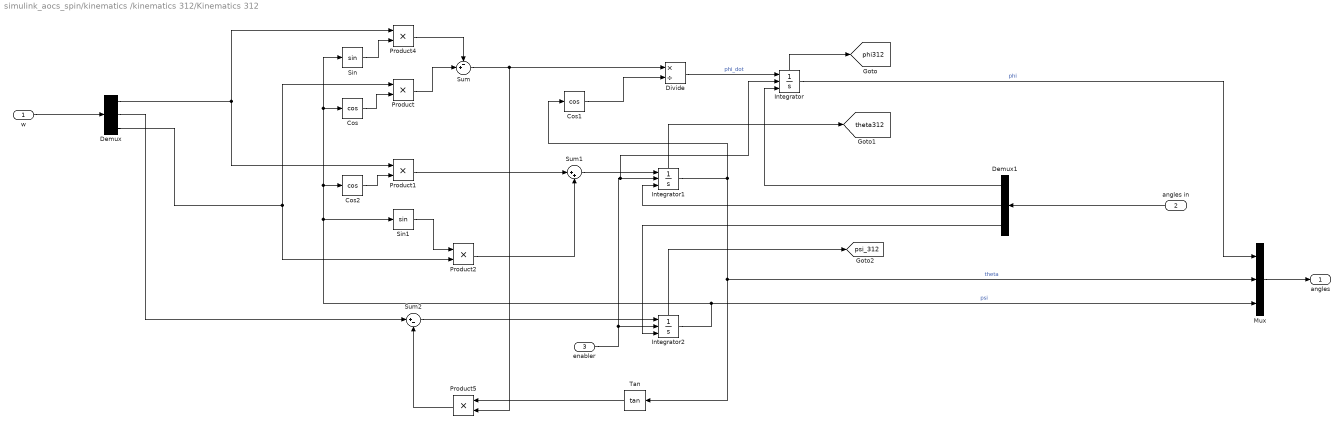
== system simulink_aocs_spin/kinematics /kinematics 312/Kinematics 312 ==
  w : Inport
  angles in : Inport  Port=2
  enabler : Inport  Port=3
  Cos : Trigonometry  Operator=cos
  Cos1 : Trigonometry  Operator=cos
  Cos2 : Trigonometry  Operator=cos
  Demux : Demux  Outputs=3
  Demux1 : Demux  Outputs=3
  Divide : Product  Inputs=*/
  Integrator : Integrator  ExternalReset=rising  InitialConditionSource=external  ShowStatePort=on
  Integrator1 : Integrator  ExternalReset=rising  InitialConditionSource=external  ShowStatePort=on
  Integrator2 : Integrator  ExternalReset=rising  InitialConditionSource=external  ShowStatePort=on  IgnoreLimit=on  ZeroCross=off
  Mux : Mux  Inputs=3
  Product{,1..2,4..5} (5 alike) : Product
  Sin : Trigonometry
  Sin1 : Trigonometry
  Sum : Sum  Inputs=-+|
  Sum1 : Sum  Inputs=|++
  Sum2 : Sum  Inputs=|+-
  Tan : Trigonometry  Operator=tan
  angles : Outport
  tag scope: phi312=global, psi_312=global, theta312=global
  wires:
  Integrator/1 -> Mux/1  "phi"
  Integrator1/1 -> Tan/1, Mux/2, Cos1/1  "theta"
  Integrator2/1 -> Sin/1, Cos/1, Cos2/1, Sin1/1, Mux/3  "psi"
  Cos/1 -> Product/2
  Demux/3 -> Product/1, Product2/2
  Product/1 -> Sum/2
  Sin/1 -> Product4/2
  Demux/1 -> Product4/1, Product1/1
  Cos1/1 -> Divide/2
  Divide/1 -> Integrator/1  "phi_dot"
  Cos2/1 -> Product1/2
  Product1/1 -> Sum1/1
  Sin1/1 -> Product2/1
  Product2/1 -> Sum1/2
  Sum1/1 -> Integrator1/1
  Product4/1 -> Sum/1
  Sum2/1 -> Integrator2/1
  Sum/1 -> Divide/1, Product5/2
  Tan/1 -> Product5/1
  Product5/1 -> Sum2/2
  Demux/2 -> Sum2/1
  w/1 -> Demux/1
  Mux/1 -> angles/1
  angles in/1 -> Demux1/1
  Demux1/1 -> Integrator/3
  Demux1/2 -> Integrator1/3
  Demux1/3 -> Integrator2/3
  enabler/1 -> Integrator/2, Integrator1/2, Integrator2/2
  Integrator/State -> [phi312]
  Integrator1/State -> [theta312]
  Integrator2/State -> [psi_312]

== system simulink_aocs_spin/kinematics /kinematics 312/Rotation 312 matrix1 ==
  angles : Inport
  A312 conc : Concatenate  NumInputs=3  Mode=Multidimensional array  ConcatenateDimension=2
  Demux : Demux  Outputs=3
  Subsystem : Subsystem
  Subsystem1 : Subsystem
  Subsystem2 : Subsystem
  column 1 : Subsystem
  column 2 : Subsystem
  column 3 : Subsystem
  A312 : Outport
  wires:
  angles/1 -> Demux/1
  Subsystem1/1(cos) -> column 2/3(theta), column 3/1(theta), column 1/3(theta)
  Subsystem/2(sin) -> column 1/2(phi2), column 2/2(phi2)
  Subsystem1/2(sin) -> column 3/2(theta2), column 1/4(theta2), column 2/4(theta2)
  Subsystem2/1(cos) -> column 2/5(psi), column 1/5(psi), column 3/3(psi)
  column 2/1(Out1) -> A312 conc/2
  Demux/2 -> Subsystem1/1(angle)
  Subsystem2/2(sin) -> column 1/6(psi2), column 2/6(psi2), column 3/4(psi2)
  Demux/3 -> Subsystem2/1(angle)
  column 1/1(Out1) -> A312 conc/1
  column 3/1(Out1) -> A312 conc/3
  Demux/1 -> Subsystem/1(angle)
  Subsystem/1(cos) -> column 1/1(phi), column 2/1(phi)
  A312 conc/1 -> A312/1

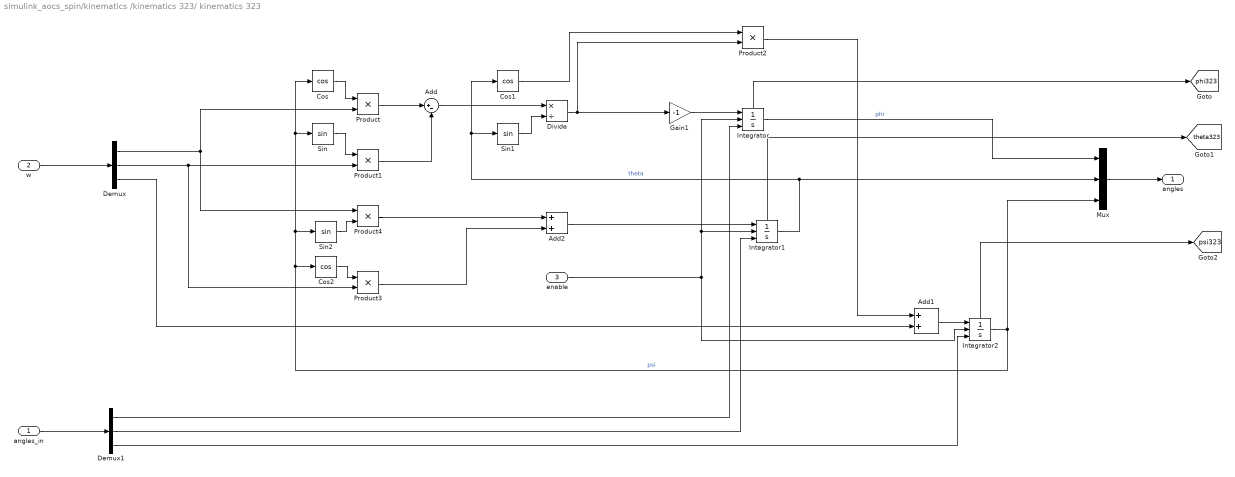
== system simulink_aocs_spin/kinematics /kinematics 323/ kinematics 323 ==
  angles_in : Inport
  w : Inport  Port=2
  enable : Inport  Port=3
  Add : Sum  Inputs=|+-
  Add1 : Sum
  Add2 : Sum
  Cos : Trigonometry  Operator=cos
  Cos1 : Trigonometry  Operator=cos
  Cos2 : Trigonometry  Operator=cos
  Demux : Demux  Outputs=3
  Demux1 : Demux  Outputs=3
  Divide : Product  Inputs=*/
  Gain1 : Gain  Gain=-1
  Integrator : Integrator  ExternalReset=rising  InitialConditionSource=external  ShowStatePort=on
  Integrator1 : Integrator  ExternalReset=rising  InitialConditionSource=external  ShowStatePort=on
  Integrator2 : Integrator  ExternalReset=rising  InitialConditionSource=external  ShowStatePort=on
  Mux : Mux  Inputs=3
  Product{,1..4} (5 alike) : Product
  Sin : Trigonometry
  Sin1 : Trigonometry
  Sin2 : Trigonometry
  angles : Outport
  tag scope: phi323=global, psi323=global, theta323=global
  wires:
  w/1 -> Demux/1
  Integrator2/1 -> Mux/3, Cos/1, Sin/1, Sin2/1, Cos2/1  "psi"
  Integrator1/1 -> Mux/2, Sin1/1, Cos1/1  "theta"
  Integrator/1 -> Mux/1  "phi"
  Demux/1 -> Product4/1, Product/2
  Cos/1 -> Product/1
  Product/1 -> Add/1
  Demux/2 -> Product3/2, Product1/2
  Sin/1 -> Product1/1
  Product1/1 -> Add/2
  Add/1 -> Divide/1
  Sin1/1 -> Divide/2
  Divide/1 -> Gain1/1, Product2/2
  Gain1/1 -> Integrator/1
  Cos1/1 -> Product2/1
  Demux/3 -> Add1/2
  Product2/1 -> Add1/1
  Add1/1 -> Integrator2/1
  Demux1/3 -> Integrator2/3
  Demux1/1 -> Integrator/3
  Cos2/1 -> Product3/1
  Sin2/1 -> Product4/2
  Product4/1 -> Add2/1
  Product3/1 -> Add2/2
  Add2/1 -> Integrator1/1
  Demux1/2 -> Integrator1/3
  Mux/1 -> angles/1
  angles_in/1 -> Demux1/1
  enable/1 -> Integrator/2, Integrator1/2, Integrator2/2
  Integrator/State -> [phi323]
  Integrator1/State -> [theta323]
  Integrator2/State -> [psi323]

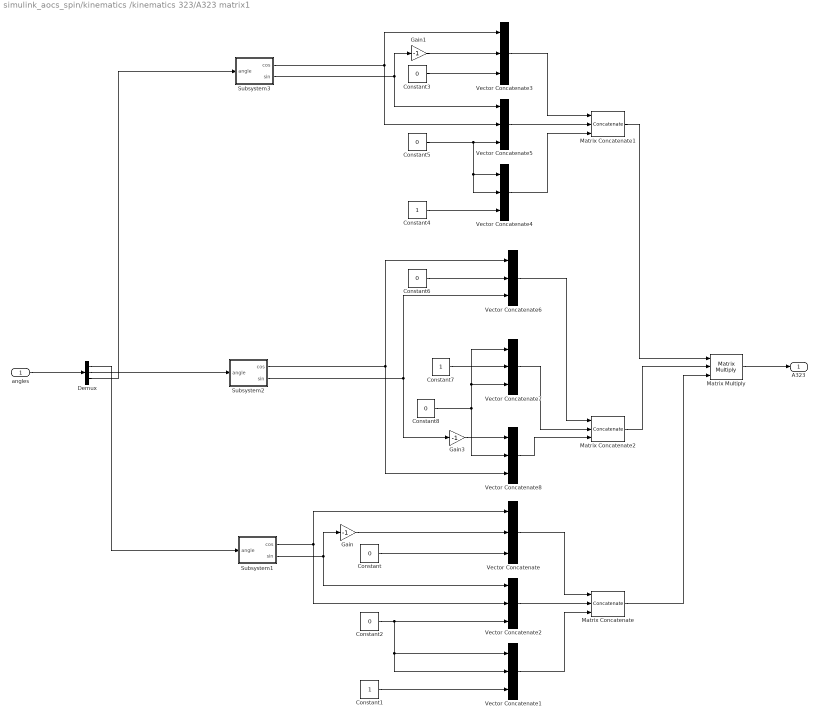
== system simulink_aocs_spin/kinematics /kinematics 323/A323 matrix1 ==
  angles : Inport
  Constant{,2..3,5..6,8} (6 alike) : Constant  Value=0
  Constant1 : Constant
  Constant4 : Constant
  Constant7 : Constant
  Demux : Demux  Outputs=3
  Gain : Gain  Gain=-1
  Gain1 : Gain  Gain=-1
  Gain3 : Gain  Gain=-1
  Matrix Concatenate : Concatenate  NumInputs=3  Mode=Multidimensional array  ConcatenateDimension=2
  Matrix Concatenate1 : Concatenate  NumInputs=3  Mode=Multidimensional array  ConcatenateDimension=2
  Matrix Concatenate2 : Concatenate  NumInputs=3  Mode=Multidimensional array  ConcatenateDimension=2
  Matrix Multiply : Product  Inputs=3  Multiplication=Matrix(*)
  Subsystem1 : Subsystem
  Subsystem2 : Subsystem
  Subsystem3 : Subsystem
  Vector Concatenate{,1..8} (9 alike) : Concatenate  NumInputs=3
  A323 : Outport
  wires:
  angles/1 -> Demux/1
  Demux/1 -> Subsystem1/1(angle)
  Demux/2 -> Subsystem2/1(angle)
  Demux/3 -> Subsystem3/1(angle)
  Gain3/1 -> Vector Concatenate8/1
  Constant8/1 -> Vector Concatenate8/2, Vector Concatenate7/3, Vector Concatenate7/1
  Constant7/1 -> Vector Concatenate7/2
  Subsystem2/2(sin) -> Gain3/1, Vector Concatenate6/3
  Constant6/1 -> Vector Concatenate6/2
  Subsystem2/1(cos) -> Vector Concatenate6/1, Vector Concatenate8/3
  Vector Concatenate8/1 -> Matrix Concatenate2/3
  Vector Concatenate7/1 -> Matrix Concatenate2/2
  Vector Concatenate6/1 -> Matrix Concatenate2/1
  Matrix Multiply/1 -> A323/1
  Matrix Concatenate1/1 -> Matrix Multiply/1
  Matrix Concatenate/1 -> Matrix Multiply/3
  Matrix Concatenate2/1 -> Matrix Multiply/2
  Subsystem3/2(sin) -> Gain1/1, Vector Concatenate5/1
  Subsystem3/1(cos) -> Vector Concatenate5/2, Vector Concatenate3/1
  Constant4/1 -> Vector Concatenate4/3
  Gain1/1 -> Vector Concatenate3/2
  Constant3/1 -> Vector Concatenate3/3
  Constant5/1 -> Vector Concatenate4/2, Vector Concatenate4/1, Vector Concatenate5/3
  Vector Concatenate3/1 -> Matrix Concatenate1/1
  Vector Concatenate5/1 -> Matrix Concatenate1/2
  Vector Concatenate4/1 -> Matrix Concatenate1/3
  Vector Concatenate1/1 -> Matrix Concatenate/3
  Vector Concatenate2/1 -> Matrix Concatenate/2
  Vector Concatenate/1 -> Matrix Concatenate/1
  Constant2/1 -> Vector Concatenate2/3, Vector Concatenate1/2, Vector Concatenate1/1
  Constant/1 -> Vector Concatenate/3
  Gain/1 -> Vector Concatenate/2
  Constant1/1 -> Vector Concatenate1/3
  Subsystem1/1(cos) -> Vector Concatenate/1, Vector Concatenate2/2
  Subsystem1/2(sin) -> Vector Concatenate2/1, Gain/1

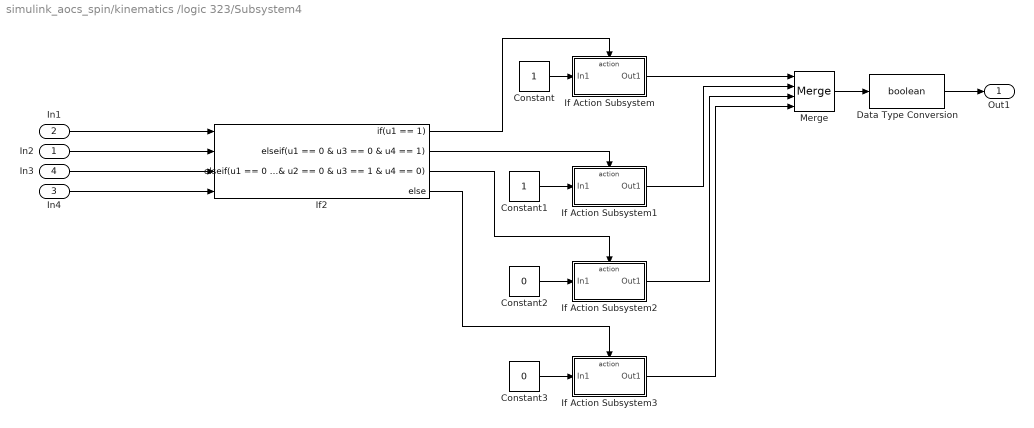
== system simulink_aocs_spin/kinematics /logic 323/Subsystem4 ==
  In2 : Inport
  In1 : Inport  Port=2
  In4 : Inport  Port=3
  In3 : Inport  Port=4
  Constant : Constant
  Constant1 : Constant
  Constant2 : Constant  Value=0
  Constant3 : Constant  Value=0
  Data Type Conversion : DataTypeConversion  OutDataTypeStr=boolean  SaturateOnIntegerOverflow=off  RndMeth=Floor
  If Action Subsystem : Subsystem  TreatAsAtomicUnit=on
  If Action Subsystem1 : Subsystem  TreatAsAtomicUnit=on
  If Action Subsystem2 : Subsystem  TreatAsAtomicUnit=on
  If Action Subsystem3 : Subsystem  TreatAsAtomicUnit=on
  If2 : If  NumInputs=4  IfExpression=u1 == 1  ElseIfExpressions=u1 == 0 & u3 == 0 & u4 == 1, u1 == 0 & u2 == 0 & u3 == 1 & u4 == 0
  Merge : Merge  Inputs=4
  Out1 : Outport
  wires:
  If2/1 -> If Action Subsystem/Action
  If2/2 -> If Action Subsystem1/Action
  If2/3 -> If Action Subsystem2/Action
  If2/4 -> If Action Subsystem3/Action
  Constant/1 -> If Action Subsystem/1(In1)
  Constant1/1 -> If Action Subsystem1/1(In1)
  Constant2/1 -> If Action Subsystem2/1(In1)
  Constant3/1 -> If Action Subsystem3/1(In1)
  If Action Subsystem/1(Out1) -> Merge/1
  If Action Subsystem1/1(Out1) -> Merge/2
  If Action Subsystem2/1(Out1) -> Merge/3
  If Action Subsystem3/1(Out1) -> Merge/4
  Merge/1 -> Data Type Conversion/1
  Data Type Conversion/1 -> Out1/1
  In1/1 -> If2/1
  In2/1 -> If2/2
  In3/1 -> If2/3
  In4/1 -> If2/4

== system simulink_aocs_spin/kinematics /312 Logic/Subsystem3/If Action Subsystem ==
  In1 : Inport
  Action Port : ActionPort  ActionPortLabel=if(u1 == 1)
  Out1 : Outport
  wires:
  In1/1 -> Out1/1

== system simulink_aocs_spin/kinematics /312 Logic/Subsystem3/If Action Subsystem1 ==
  In1 : Inport
  Action Port : ActionPort  ActionPortLabel=elseif(u1 == 0 & u2 == 1 & u3 == 1)
  Out1 : Outport
  wires:
  In1/1 -> Out1/1

== system simulink_aocs_spin/kinematics /312 Logic/Subsystem3/If Action Subsystem2 ==
  In1 : Inport
  Action Port : ActionPort  ActionPortLabel=elseif( u1 == 0 & u2 == 1 & u3 == 0)
  Out1 : Outport
  wires:
  In1/1 -> Out1/1

== system simulink_aocs_spin/kinematics /312 Logic/Subsystem3/If Action Subsystem3 ==
  In1 : Inport
  Action Port : ActionPort  ActionPortLabel=else
  Out1 : Outport
  wires:
  In1/1 -> Out1/1

== system simulink_aocs_spin/kinematics /angles 312 new/A323 matrix/Subsystem1 ==
  angle : Inport
  Cos : Trigonometry  Operator=cos
  Sin : Trigonometry
  cos : Outport
  sin : Outport  Port=2
  wires:
  angle/1 -> Cos/1, Sin/1
  Sin/1 -> sin/1
  Cos/1 -> cos/1

== system simulink_aocs_spin/kinematics /angles 312 new/A323 matrix/Subsystem2 ==
  angle : Inport
  Cos : Trigonometry  Operator=cos
  Sin : Trigonometry
  cos : Outport
  sin : Outport  Port=2
  wires:
  angle/1 -> Cos/1, Sin/1
  Sin/1 -> sin/1
  Cos/1 -> cos/1

== system simulink_aocs_spin/kinematics /angles 312 new/A323 matrix/Subsystem3 ==
  angle : Inport
  Cos : Trigonometry  Operator=cos
  Sin : Trigonometry
  cos : Outport
  sin : Outport  Port=2
  wires:
  Cos/1 -> cos/1
  Sin/1 -> sin/1
  angle/1 -> Sin/1, Cos/1

== system simulink_aocs_spin/kinematics /angles 323 new/Rotation 312 matrix2/Subsystem ==
  angle : Inport
  Cos : Trigonometry  Operator=cos
  Sin : Trigonometry
  cos : Outport
  sin : Outport  Port=2
  wires:
  Cos/1 -> cos/1
  Sin/1 -> sin/1
  angle/1 -> Sin/1, Cos/1

== system simulink_aocs_spin/kinematics /angles 323 new/Rotation 312 matrix2/Subsystem1 ==
  angle : Inport
  Cos : Trigonometry  Operator=cos
  Sin : Trigonometry
  cos : Outport
  sin : Outport  Port=2
  wires:
  angle/1 -> Cos/1, Sin/1
  Sin/1 -> sin/1
  Cos/1 -> cos/1

== system simulink_aocs_spin/kinematics /angles 323 new/Rotation 312 matrix2/Subsystem2 ==
  angle : Inport
  Cos : Trigonometry  Operator=cos
  Sin : Trigonometry
  cos : Outport
  sin : Outport  Port=2
  wires:
  Cos/1 -> cos/1
  Sin/1 -> sin/1
  angle/1 -> Sin/1, Cos/1

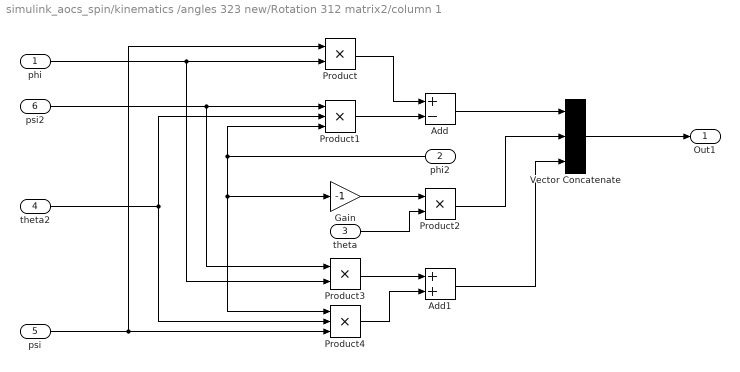
== system simulink_aocs_spin/kinematics /angles 323 new/Rotation 312 matrix2/column 1 ==
  phi : Inport
  phi2 : Inport  Port=2
  theta : Inport  Port=3
  theta2 : Inport  Port=4
  psi : Inport  Port=5
  psi2 : Inport  Port=6
  Add : Sum  Inputs=+-
  Add1 : Sum
  Gain : Gain  Gain=-1
  Product : Product
  Product1 : Product  Inputs=3
  Product2 : Product
  Product3 : Product
  Product4 : Product  Inputs=3
  Vector Concatenate : Concatenate  NumInputs=3
  Out1 : Outport
  wires:
  Add1/1 -> Vector Concatenate/3
  psi/1 -> Product/1, Product4/3
  theta2/1 -> Product4/2, Product1/2
  phi2/1 -> Product4/1, Gain/1, Product1/3
  psi2/1 -> Product3/1, Product1/1
  Gain/1 -> Product2/1
  phi/1 -> Product3/2, Product/2
  Product3/1 -> Add1/1
  Product1/1 -> Add/2
  Product2/1 -> Vector Concatenate/2
  Vector Concatenate/1 -> Out1/1
  Product/1 -> Add/1
  Add/1 -> Vector Concatenate/1
  Product4/1 -> Add1/2
  theta/1 -> Product2/2

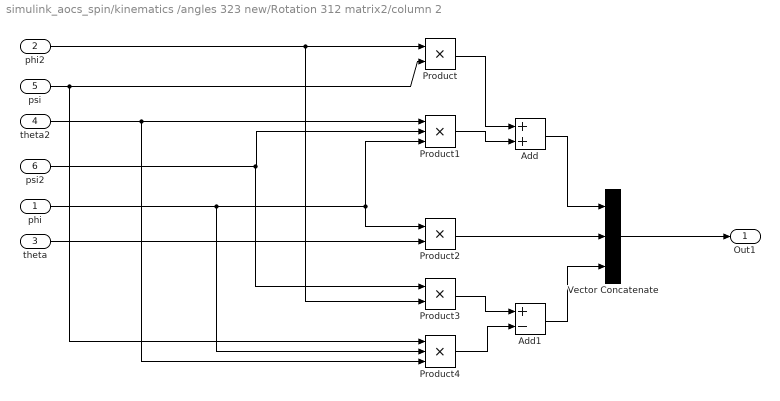
== system simulink_aocs_spin/kinematics /angles 323 new/Rotation 312 matrix2/column 2 ==
  phi : Inport
  phi2 : Inport  Port=2
  theta : Inport  Port=3
  theta2 : Inport  Port=4
  psi : Inport  Port=5
  psi2 : Inport  Port=6
  Add : Sum
  Add1 : Sum  Inputs=+-
  Product : Product
  Product1 : Product  Inputs=3
  Product2 : Product
  Product3 : Product
  Product4 : Product  Inputs=3
  Vector Concatenate : Concatenate  NumInputs=3
  Out1 : Outport
  wires:
  Add1/1 -> Vector Concatenate/3
  theta2/1 -> Product4/3, Product1/1
  phi/1 -> Product4/2, Product2/1, Product1/3
  Product3/1 -> Add1/1
  Add/1 -> Vector Concatenate/1
  Product4/1 -> Add1/2
  Product2/1 -> Vector Concatenate/2
  Product1/1 -> Add/2
  phi2/1 -> Product3/2, Product/1
  Product/1 -> Add/1
  Vector Concatenate/1 -> Out1/1
  theta/1 -> Product2/2
  psi/1 -> Product4/1, Product/2
  psi2/1 -> Product3/1, Product1/2

== system simulink_aocs_spin/kinematics /angles 323 new/Rotation 312 matrix2/column 3 ==
  theta : Inport
  theta2 : Inport  Port=2
  psi : Inport  Port=3
  psi2 : Inport  Port=4
  Gain : Gain  Gain=-1
  Product : Product
  Product1 : Product
  Vector Concatenate : Concatenate  NumInputs=3
  Out1 : Outport
  wires:
  Product/1 -> Gain/1
  theta/1 -> Product1/1, Product/2
  Gain/1 -> Vector Concatenate/1
  psi2/1 -> Product/1
  Product1/1 -> Vector Concatenate/3
  theta2/1 -> Vector Concatenate/2
  psi/1 -> Product1/2
  Vector Concatenate/1 -> Out1/1

== system simulink_aocs_spin/kinematics /kinematics 312/Rotation 312 matrix1/Subsystem ==
  angle : Inport
  Cos : Trigonometry  Operator=cos
  Sin : Trigonometry
  cos : Outport
  sin : Outport  Port=2
  wires:
  angle/1 -> Cos/1, Sin/1
  Sin/1 -> sin/1
  Cos/1 -> cos/1

== system simulink_aocs_spin/kinematics /kinematics 312/Rotation 312 matrix1/Subsystem1 ==
  angle : Inport
  Cos : Trigonometry  Operator=cos
  Sin : Trigonometry
  cos : Outport
  sin : Outport  Port=2
  wires:
  Cos/1 -> cos/1
  Sin/1 -> sin/1
  angle/1 -> Sin/1, Cos/1

== system simulink_aocs_spin/kinematics /kinematics 312/Rotation 312 matrix1/Subsystem2 ==
  angle : Inport
  Cos : Trigonometry  Operator=cos
  Sin : Trigonometry
  cos : Outport
  sin : Outport  Port=2
  wires:
  angle/1 -> Cos/1, Sin/1
  Sin/1 -> sin/1
  Cos/1 -> cos/1

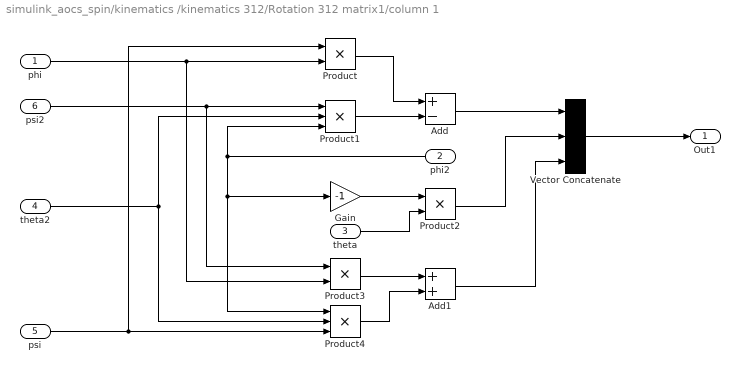
== system simulink_aocs_spin/kinematics /kinematics 312/Rotation 312 matrix1/column 1 ==
  phi : Inport
  phi2 : Inport  Port=2
  theta : Inport  Port=3
  theta2 : Inport  Port=4
  psi : Inport  Port=5
  psi2 : Inport  Port=6
  Add : Sum  Inputs=+-
  Add1 : Sum
  Gain : Gain  Gain=-1
  Product : Product
  Product1 : Product  Inputs=3
  Product2 : Product
  Product3 : Product
  Product4 : Product  Inputs=3
  Vector Concatenate : Concatenate  NumInputs=3
  Out1 : Outport
  wires:
  theta/1 -> Product2/2
  Product4/1 -> Add1/2
  Add/1 -> Vector Concatenate/1
  Product/1 -> Add/1
  Vector Concatenate/1 -> Out1/1
  Product2/1 -> Vector Concatenate/2
  Product1/1 -> Add/2
  Product3/1 -> Add1/1
  phi/1 -> Product/2, Product3/2
  Gain/1 -> Product2/1
  psi2/1 -> Product1/1, Product3/1
  phi2/1 -> Product1/3, Gain/1, Product4/1
  theta2/1 -> Product1/2, Product4/2
  psi/1 -> Product4/3, Product/1
  Add1/1 -> Vector Concatenate/3

== system simulink_aocs_spin/kinematics /kinematics 312/Rotation 312 matrix1/column 2 ==
  phi : Inport
  phi2 : Inport  Port=2
  theta : Inport  Port=3
  theta2 : Inport  Port=4
  psi : Inport  Port=5
  psi2 : Inport  Port=6
  Add : Sum
  Add1 : Sum  Inputs=+-
  Product : Product
  Product1 : Product  Inputs=3
  Product2 : Product
  Product3 : Product
  Product4 : Product  Inputs=3
  Vector Concatenate : Concatenate  NumInputs=3
  Out1 : Outport
  wires:
  psi2/1 -> Product1/2, Product3/1
  psi/1 -> Product/2, Product4/1
  theta/1 -> Product2/2
  Vector Concatenate/1 -> Out1/1
  Product/1 -> Add/1
  phi2/1 -> Product/1, Product3/2
  Product1/1 -> Add/2
  Product2/1 -> Vector Concatenate/2
  Product4/1 -> Add1/2
  Add/1 -> Vector Concatenate/1
  Product3/1 -> Add1/1
  phi/1 -> Product1/3, Product2/1, Product4/2
  theta2/1 -> Product1/1, Product4/3
  Add1/1 -> Vector Concatenate/3

== system simulink_aocs_spin/kinematics /kinematics 312/Rotation 312 matrix1/column 3 ==
  theta : Inport
  theta2 : Inport  Port=2
  psi : Inport  Port=3
  psi2 : Inport  Port=4
  Gain : Gain  Gain=-1
  Product : Product
  Product1 : Product
  Vector Concatenate : Concatenate  NumInputs=3
  Out1 : Outport
  wires:
  Vector Concatenate/1 -> Out1/1
  psi/1 -> Product1/2
  theta2/1 -> Vector Concatenate/2
  Product1/1 -> Vector Concatenate/3
  psi2/1 -> Product/1
  Gain/1 -> Vector Concatenate/1
  theta/1 -> Product/2, Product1/1
  Product/1 -> Gain/1

== system simulink_aocs_spin/kinematics /kinematics 323/A323 matrix1/Subsystem1 ==
  angle : Inport
  Cos : Trigonometry  Operator=cos
  Sin : Trigonometry
  cos : Outport
  sin : Outport  Port=2
  wires:
  Cos/1 -> cos/1
  Sin/1 -> sin/1
  angle/1 -> Sin/1, Cos/1

== system simulink_aocs_spin/kinematics /kinematics 323/A323 matrix1/Subsystem2 ==
  angle : Inport
  Cos : Trigonometry  Operator=cos
  Sin : Trigonometry
  cos : Outport
  sin : Outport  Port=2
  wires:
  Cos/1 -> cos/1
  Sin/1 -> sin/1
  angle/1 -> Sin/1, Cos/1

== system simulink_aocs_spin/kinematics /kinematics 323/A323 matrix1/Subsystem3 ==
  angle : Inport
  Cos : Trigonometry  Operator=cos
  Sin : Trigonometry
  cos : Outport
  sin : Outport  Port=2
  wires:
  angle/1 -> Cos/1, Sin/1
  Sin/1 -> sin/1
  Cos/1 -> cos/1

== system simulink_aocs_spin/kinematics /logic 323/Subsystem4/If Action Subsystem ==
  In1 : Inport
  Action Port : ActionPort  ActionPortLabel=if(u1 == 1)
  Out1 : Outport
  wires:
  In1/1 -> Out1/1

== system simulink_aocs_spin/kinematics /logic 323/Subsystem4/If Action Subsystem1 ==
  In1 : Inport
  Action Port : ActionPort  ActionPortLabel=elseif(u1 == 0 & u3 == 0 & u4 == 1)
  Out1 : Outport
  wires:
  In1/1 -> Out1/1

== system simulink_aocs_spin/kinematics /logic 323/Subsystem4/If Action Subsystem2 ==
  In1 : Inport
  Action Port : ActionPort  ActionPortLabel=elseif( u1 == 0 & u2 == 0 & u3 == 1 & u4 == 0)
  Out1 : Outport
  wires:
  In1/1 -> Out1/1

== system simulink_aocs_spin/kinematics /logic 323/Subsystem4/If Action Subsystem3 ==
  In1 : Inport
  Action Port : ActionPort  ActionPortLabel=else
  Out1 : Outport
  wires:
  In1/1 -> Out1/1
